simulink model "WindFarmGFMControlFast"  (R2023a)
settings: Solver=VariableStepAuto  StartTime=0.0  StopTime=Tsim  FixedStep=Ts  MaxStep=1  MinStep=Ts  RelTol=1e-3
PreLoadFcn:
  | run('WindFarmGFMControlParametersFast.m')
undefined symbols (not defined in the file): DiscIntNeverNeededParam, feeder, frt, gGFM, grid, line, loads, lvrt, mGFM, pmsm, time, Ts, windController, windTransformer, windTurbine
libraries: ee_lib x21, nesl_utility x14, eeGeneralControl x4, fl_lib x3, spsLeadLagFilterLib x2, eeTransforms x2, eePowerMeasurement x1, eeSinusoidalMeasurementV2 x1
(part 1 of 2)
settings Model: SimulationMode=accelerator  Creator=rajarshd  LastModifiedBy=rajarshd
settings SolverCC: MaxConsecutiveZCs=1  ZeroCrossAlgorithm=Adaptive  AutoInsertRateTranBlk=on  DecoupledContinuousIntegration=on
settings DataIOCC: ExternalInput=getinputstruct(op)  InitialState=getstatestruct(op)  SaveFormat=StructureWithTime  SaveOutput=off  DSMLogging=off  SignalLoggingName=logsWindGFMControl
settings OptimizationCC: ReuseModelBlockBuffer=off
settings DebuggingCC: IgnoredZcDiagnostic=none
settings ModelReferenceCC: EnableRefExpFcnMdlSchedulingChecks=on  EnableParallelModelReferenceBuilds=on  ParallelModelReferenceMATLABWorkerInit=Load Top Model
settings SimscapeCC: ExplicitSolverDiagnosticOptions=none  SimscapeLogType=all  SimscapeLogSimulationStatistics=on  SimscapeLogName=simlogWindFarmGFMControl  SimscapeOperatingPoint=op

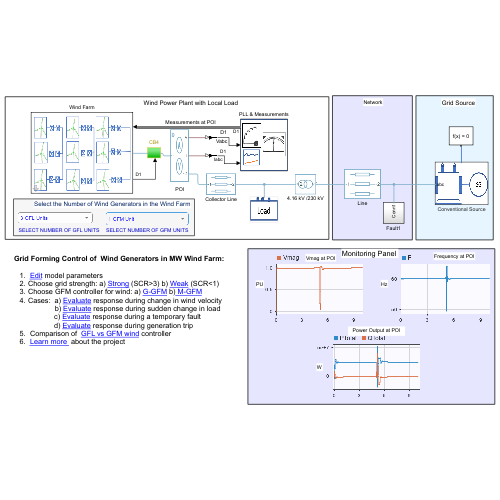
[thumbnail: Simulink's stored preview of the top-level diagram]
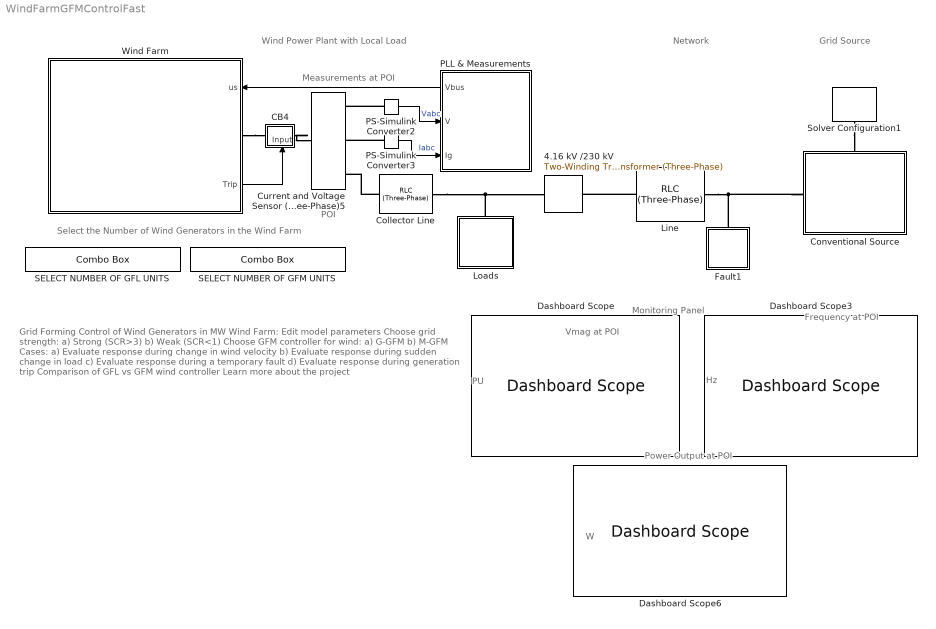
== system WindFarmGFMControlFast ==
  note: Select the Number of Wind Generators in the Wind Farm
  note: POI
  note: Measurements at POI
  note: Grid Source
  note: Wind Power Plant with Local Load
  note: Vmag at POI
  note: Frequency at POI
  note: Hz
  note: PU
  note: Grid Forming Control of Wind Generators in MW Wind Farm:
      |
      | Edit model parameters
      | Choose grid strength: a) Strong (SCR>3) b) Weak (SCR<1)
      | Choose GFM controller for wind: a) G-GFM b) M-GFM
      | Cases: a) Evaluate response during change in wind velocity
      | b) Evaluate response during sudden change in load
      | c) Evaluate response during a temporary fault
      | d) Evaluate response during generation trip
      | Comparison of GFL vs GFM wind controller
      | Learn more about the project
  note: Monitoring Panel
  note: Power Output at POI
  note: Network
  note: W
  4.16 kV /230 kV : ee_lib/Passive/Transformers/Two-Winding Transformer (Three-Phase)  SRated=windTransformer.va A*V  FRated=grid.frequency Hz  Winding1Connection=ee.enum.windingconnection.Yg  VRated1=windTransformer.hv V  Winding2Connection=ee.enum.windingconnection.Yg  VRated2=windTransformer.lv V  CoreType=ee.enum.coretype.threelimb  pu_Rw1=windTransformer.windingResistance/2  pu_Rw2=windTransformer.windingResistance/2  leakage_reactance_option=ee.enum.transformer_leakage.include  pu_Xl1=windTransformer.windingLekageReactance/2  pu_Xl2=windTransformer.windingLekageReactance/2  magnetizing_resistance_option=ee.enum.transformer_magnetizingResistance.exclude  pu_Rm=500  magnetizing_reactance_option=ee.enum.transformer_magnetizingReactance.exclude  saturation_option=ee.enum.transformer_saturation.exclude  pu_Xm=500  current_data=[0, .002, 1, 2]  magnetic_flux_data=[0, 1.2, 1.5, 1.51]  pu_X0=windTransformer.zeroSequenceReactance  i1_specify=off  i1_priority=None  i1=[0, 0, 0] A  i1_nominal_specify=off  i1_nominal_unit=A  i1_nominal_value=1  i2_specify=off  i2_priority=None  i2=[0, 0, 0] A  i2_nominal_specify=off  i2_nominal_unit=A  i2_nominal_value=1  phi_specify=off  phi_priority=None  phi=[0, 0, 0]  phi_nominal_specify=off  phi_nominal_unit=1  phi_nominal_value=1  power_dissipated_specify=off  power_dissipated_priority=None  power_dissipated=0 W  power_dissipated_nominal_specify=off  power_dissipated_nominal_unit=W  power_dissipated_nominal_value=1
      settings: InternalSimscapePortConfiguration="{\"Bottom\":[],\"Left\":[{\"id\":\"N1\",\"label\":\"~1\",\"type\":\"foundation.electrical.three_phase\"}],\"Right\":[{\"id\":\"N2\",\"label\":\"~2\",\"type\":\"foundation.electrical.three_phase\"}],\"Top\":[]}"
  CB4 : Subsystem
      settings: PortSchema="{\"entries\":[{\"content\":{\"sides\":[{\"content\":{\"connectorIds\":[\"LConn1\"]},\"type\":\"ConnectorPlacement.EquallySpacedRectSide\",\"uuid\":\"67c0f727-7c15-41c9-98df-b3c7d57498ed\"},{\"content\":{\"connectorIds\":[\"RConn1\"],\"side\":\"RIGHT\"},\"type\":\"ConnectorPlacement.EquallySpacedRectSide\",\"uuid\":\"7fc39429-ba61-416d-b42b-93e81eb2f426\"},{\"content\":{\"side\":\"TOP\"},\"type\":\"ConnectorPlacement.EquallySpacedRectSide\",\"uuid\":\"c6dd9263-b57a-4cff-a218-af99f2798f29\"},{\"content\":{\"connectorIds\":[\"In1\"],\"side\":\"BOTTOM\"},\"type\":\"ConnectorPlacement.EquallySpacedRectSide\",\"uuid\":\"e2a2ba44-d59d-4e27-adf1-3f94e828ca78\"}]},\"type\":\"ConnectorPlacement.EquallySpacedConnector\",\"uuid\":\"b349a99b-c902-4df9-9c99-34841afb28dd\"}],\"packageUris\":[\"http://schema.mathworks.com/mf0/Connector/R2020b\"],\"version\":\"1.0\"}"
  Collector Line : ee_lib/Passive/RLC Assemblies/RLC (Three-Phase)  component_structure=ee.enum.rlc.structure.SeriesRL  R=feeder.r*feeder.length Ohm  L=feeder.l*feeder.length H  C=1e-6 F  R_parasitic=0 Ohm  G_parasitic=0 1/Ohm  IL_specify=off  IL_priority=High  IL=[0, 0, 0] A  IL_nominal_specify=off  IL_nominal_unit=A  IL_nominal_value=1  VC_specify=off  VC_priority=High  VC=[0, 0, 0] V  VC_nominal_specify=off  VC_nominal_unit=V  VC_nominal_value=1
      settings: InternalSimscapePortConfiguration="{\"Bottom\":[],\"Left\":[{\"id\":\"N1\",\"label\":\"~1\",\"type\":\"foundation.electrical.three_phase\"}],\"Right\":[{\"id\":\"N2\",\"label\":\"~2\",\"type\":\"foundation.electrical.three_phase\"}],\"Top\":[]}"
  Conventional Source : Subsystem
      settings: PortSchema="{\"entries\":[{\"content\":{\"sides\":[{\"content\":{\"connectorIds\":[\"LConn1\"]},\"type\":\"ConnectorPlacement.EquallySpacedRectSide\",\"uuid\":\"88e24179-6079-4110-b6c8-07285d357c8a\"},{\"content\":{\"connectorIds\":[],\"side\":\"RIGHT\"},\"type\":\"ConnectorPlacement.EquallySpacedRectSide\",\"uuid\":\"8f4b6582-111e-4598-90a5-fa5f81c444ee\"},{\"content\":{\"connectorIds\":[\"LConn2\"],\"side\":\"TOP\"},\"type\":\"ConnectorPlacement.EquallySpacedRectSide\",\"uuid\":\"53212e71-0f3c-4549-bc92-047e88eae9b6\"},{\"content\":{\"connectorIds\":[],\"side\":\"BOTTOM\"},\"type\":\"ConnectorPlacement.EquallySpacedRectSide\",\"uuid\":\"0193069a-d0a5-4b89-8f2a-3f6fb986b7f7\"}]},\"type\":\"ConnectorPlacement.EquallySpacedConnector\",\"uuid\":\"b2543555-7807-483c-9e73-a2cd2a98a3a5\"}],\"packageUris\":[\"http://schema.mathworks.com/mf0/Connector/R2020b\"],\"version\":\"1.0\"}"
      mask Display: image('$imagefile'); % Use "Edit Image" on toolstrip to change.
  Current and Voltage Sensor (Three-Phase)5 : ee_lib/Sensors & Transducers/Current and Voltage Sensor (Three-Phase)  vMeasurementType=ee.enum.vmeasurement.lg  outputUnit=ee.enum.unit.pu  SRated=base.mVA A*V  VRated=base.kV V  I_specify=off  I_priority=None  I=[0, 0, 0] A  I_nominal_specify=off  I_nominal_unit=A  I_nominal_value=1  V_specify=off  V_priority=None  V=[0, 0, 0] V  V_nominal_specify=off  V_nominal_unit=V  V_nominal_value=1
      settings: InternalSimscapePortConfiguration="{\"Bottom\":[],\"Left\":[{\"id\":\"N1\",\"label\":\"~1\",\"type\":\"foundation.electrical.three_phase\"}],\"Right\":[{\"id\":\"V_output\",\"label\":\"V\",\"type\":\"output\"},{\"id\":\"I_output\",\"label\":\"I\",\"type\":\"output\"},{\"id\":\"N2\",\"label\":\"~2\",\"type\":\"foundation.electrical.three_phase\"}],\"Top\":[]}"
  Dashboard Scope : DashboardScope  Ymin=-0.6  Ymax=1.1
  Dashboard Scope3 : DashboardScope  Ymin=50  Ymax=80
  Dashboard Scope6 : DashboardScope
  Fault1 : Subsystem
      settings: PortSchema="{\"entries\":[{\"content\":{\"sides\":[{\"content\":{},\"type\":\"ConnectorPlacement.EquallySpacedRectSide\",\"uuid\":\"8f0a92ab-8e67-482c-af4d-aec2c4f39f54\"},{\"content\":{\"side\":\"RIGHT\"},\"type\":\"ConnectorPlacement.EquallySpacedRectSide\",\"uuid\":\"ef292762-0220-4a9e-ab1f-c2e04fa471eb\"},{\"content\":{\"connectorIds\":[\"LConn1\"],\"side\":\"TOP\"},\"type\":\"ConnectorPlacement.EquallySpacedRectSide\",\"uuid\":\"ae2b4012-1172-468f-8626-eed330b859d8\"}]},\"type\":\"ConnectorPlacement.EquallySpacedConnector\",\"uuid\":\"c563c82f-8ad7-4cb2-b357-8e612dcbe120\"}],\"packageUris\":[\"http://schema.mathworks.com/mf0/Connector/R2020b\"],\"version\":\"1.0\"}"
  Line : ee_lib/Passive/RLC Assemblies/RLC (Three-Phase)  component_structure=ee.enum.rlc.structure.SeriesRL  R=line.r*line.length1 Ohm  L=line.l*line.length1 mH  C=1e-6 F  R_parasitic=0 Ohm  G_parasitic=0 1/Ohm  IL_specify=off  IL_priority=High  IL=[0, 0, 0] A  IL_nominal_specify=off  IL_nominal_unit=A  IL_nominal_value=1  VC_specify=off  VC_priority=High  VC=[0, 0, 0] V  VC_nominal_specify=off  VC_nominal_unit=V  VC_nominal_value=1
      settings: InternalSimscapePortConfiguration="{\"Bottom\":[],\"Left\":[{\"id\":\"N1\",\"label\":\"~1\",\"type\":\"foundation.electrical.three_phase\"}],\"Right\":[{\"id\":\"N2\",\"label\":\"~2\",\"type\":\"foundation.electrical.three_phase\"}],\"Top\":[]}"
  Loads : Subsystem
      mask Display: image('$imagefile'); % Use "Edit Image" on toolstrip to change.
  PLL & Measurements : Subsystem
      settings: PortSchema="{\"entries\":[{\"content\":{\"sides\":[{\"content\":{\"connectorIds\":[\"Out1\",\"In1\",\"In2\"]},\"type\":\"ConnectorPlacement.EquallySpacedRectSide\",\"uuid\":\"76485780-20fe-4fcf-8224-69648da6ed2a\"},{\"content\":{\"side\":\"RIGHT\"},\"type\":\"ConnectorPlacement.EquallySpacedRectSide\",\"uuid\":\"f19a6390-e634-42c7-8d46-4cd80cbab182\"},{\"content\":{\"side\":\"TOP\"},\"type\":\"ConnectorPlacement.EquallySpacedRectSide\",\"uuid\":\"87682f72-1844-428e-be70-ad7ca3191ee3\"}]},\"type\":\"ConnectorPlacement.EquallySpacedConnector\",\"uuid\":\"f2136b07-48ec-402b-adb3-18c0bac2157c\"}],\"packageUris\":[\"http://schema.mathworks.com/mf0/Connector/R2020b\"],\"version\":\"1.0\"}"
      mask Display: image('measurements.png'); % Use "Edit Image" on toolstrip to change.
  PS-Simulink Converter2 : nesl_utility/PS-Simulink Converter  PhysicalDomain=network_engine_domain  SubClassName=ps_output  LeftPortType=input  RightPortType=output  PseudoPeriodic=off  Frequencies=[]  VectorFormat=inherit  Unit=inherit  AffineConversion=off
  PS-Simulink Converter3 : nesl_utility/PS-Simulink Converter  PhysicalDomain=network_engine_domain  SubClassName=ps_output  LeftPortType=input  RightPortType=output  PseudoPeriodic=off  Frequencies=[]  VectorFormat=inherit  Unit=inherit  AffineConversion=off
  SELECT NUMBER OF GFL UNITS : ComboBox  LabelPosition=Hide  SelectedLabel=3 GFL Units
      settings: Values={{'1 GFL Unit', '2 GFL Units', '3 GFL Units', '4 GFL Units', '5 GFL Units', '6 GFL Units', '7 GFL Units'}, [1 2 3 4 5 6 7]}
  SELECT NUMBER OF GFM UNITS : ComboBox  LabelPosition=Hide  SelectedLabel=1 GFM Unit  Opacity=0
      settings: Values={{'1 GFM Unit', '2 GFM Units', 'No GFM Units'}, [1 2 0]}
  Solver Configuration1 : nesl_utility/Solver Configuration  PhysicalDomain=network_engine_domain  SubClassName=solver  LeftPortType=input  RightPortType=generic  Tones=[]  Harmonics=[]  SimulateNoise=off  Profile=off  UseLocalSampling=off  EnableSwitchedLinearOptims=on  FrequencyDomain=off  UseCCode=off  RelTol=0.001  AbsTol=1e-06  MinStep=1e-09  ToWorkspace=off  RevertToSquareIcSolve=off  NumHomotopyIterations=100  PhasorMode=off  PhasorModeNumHarmonics=1  ConsistencySolver=NEWTON_FTOL  IndexReductionMethod=DerivativeReplacement  DoDC=off  ResidualTolerance=1e-3  ConsistencyTolSource=GLOBAL  ConsistencyAbsTol=0.001  ConsistencyRelTol=0.001  ConsistencyTolFactor=0.001  UseLocalSolver=on  LocalSolverChoice=NE_PARTITIONING_ADVANCER  ResolveIndetEquations=on  FunctionEvalNumThread=1  LocalSolverSampleTime=T  DoFixedCost=on  MaxNonlinIter=3  MaxModeIter=2  ComputeImpulses=off  ImpulseIterations=2  LinearAlgebra=auto  LinearAlgebraNumThread=0  EquationFormulation=NE_TIME_EF  DelaysMemoryBudget=1024  AutomaticFiltering=on  FilteringTimeConstant=0.001  PartitionStorageMethod=AS_NEEDED  PartitionMemoryBudget=1024  PartitionMethod=ROBUST
  Wind Farm : Subsystem  mask{nGFL=3, nGFM=1}
      mask prompts: nGFL "Number of GFL Wind Generators"; nGFM "Number of GFM Wind Turbines"
      settings: PortSchema="{\"entries\":[{\"content\":{\"sides\":[{\"content\":{\"connectorIds\":[\"In1\",\"LConn1\",\"Out1\"]},\"type\":\"ConnectorPlacement.EquallySpacedRectSide\",\"uuid\":\"1189e956-e6f0-4ada-905a-6b9abec668a8\"},{\"content\":{\"side\":\"RIGHT\"},\"type\":\"ConnectorPlacement.EquallySpacedRectSide\",\"uuid\":\"3ddb8f28-1c9c-423f-814f-a5e5ca919d79\"},{\"content\":{\"side\":\"TOP\"},\"type\":\"ConnectorPlacement.EquallySpacedRectSide\",\"uuid\":\"c360f229-efd7-488e-97f8-90fd9e6e05d4\"},{\"content\":{\"side\":\"BOTTOM\"},\"type\":\"ConnectorPlacement.EquallySpacedRectSide\",\"uuid\":\"99811ca4-1621-4e62-9767-ce3bd58f839c\"}]},\"type\":\"ConnectorPlacement.EquallySpacedConnector\",\"uuid\":\"16843f42-9f9b-4252-a0c2-a64badb15c83\"}],\"packageUris\":[\"http://schema.mathworks.com/mf0/Connector/R2020b\"],\"version\":\"1.0\"}"
      mask TypeOptions nGFL: 1 | 2 | 3 | 4 | 5 | 6 | 7
      mask TypeOptions nGFM: 0 | 1 | 2
      mask DialogControl Control1 Prompt: This is a Wind Farm with type-4 GFL and GFM Wind Turbine Generators
      mask Display: image('$imagefile'); % Use "Edit Image" on toolstrip to change.
  wires:
  PS-Simulink Converter2/1 -> PLL & Measurements/1(V)  "Vabc"
  PS-Simulink Converter3/1 -> PLL & Measurements/2(Ig)  "Iabc"
  PLL & Measurements/1(Vbus) -> Wind Farm/1(us)
  Wind Farm/1(Trip) -> CB4/1(Input)
  connections:
  Loads/RConn1 -- Collector Line/RConn1 -- 4.16 kV /230 kV/RConn1
  PS-Simulink Converter2/LConn1 -- Current and Voltage Sensor (Three-Phase)5/RConn1
  PS-Simulink Converter3/LConn1 -- Current and Voltage Sensor (Three-Phase)5/RConn2
  Solver Configuration1/RConn1 -- Conventional Source/LConn2
  CB4/RConn1 -- Current and Voltage Sensor (Three-Phase)5/LConn1
  Conventional Source/LConn1 -- Line/RConn1 -- Fault1/LConn1
  Line/LConn1 -- 4.16 kV /230 kV/LConn1
  Wind Farm/LConn1 -- CB4/LConn1
  Collector Line/LConn1 -- Current and Voltage Sensor (Three-Phase)5/RConn3

== system WindFarmGFMControlFast/CB4 ==
  Input : Inport
  Circuit Breaker Step off3 : ee_lib/Switches & Breakers/Circuit Breaker (Three-Phase)  R_closed=0.001 Ohm  G_open=1e-4 1/Ohm  threshold=0.5 V  breaker_behavior=ee.enum.switches.breakerBehavior.zeroCrossingEnable
      settings: InternalSimscapePortConfiguration="{\"Bottom\":[],\"Left\":[{\"id\":\"vT\",\"label\":\"vT\",\"type\":\"input\"},{\"id\":\"N1\",\"label\":\"~1\",\"type\":\"foundation.electrical.three_phase\"}],\"Right\":[{\"id\":\"N2\",\"label\":\"~2\",\"type\":\"foundation.electrical.three_phase\"}],\"Top\":[]}"
  Simulink-PS Converter3 : nesl_utility/Simulink-PS Converter  PhysicalDomain=network_engine_domain  SubClassName=ps_input  LeftPortType=input  RightPortType=output  PseudoPeriodic=off  Frequencies=[]  NoiseDistribution=none  NoiseParameters=[]  Unit=1  AffineConversion=off  FilteringAndDerivatives=zero  SimscapeFilterOrder=1  InputFilterTimeConstant=0.001  UdotUserProvided=1
  Conn2 : PMIOPort  Side=Left
  Conn1 : PMIOPort  Port=2  Side=Right
  wires:
  Input/1 -> Simulink-PS Converter3/1
  connections:
  Circuit Breaker Step off3/LConn2 -- Conn2/RConn1
  Circuit Breaker Step off3/LConn1 -- Simulink-PS Converter3/RConn1
  Circuit Breaker Step off3/RConn1 -- Conn1/RConn1

== system WindFarmGFMControlFast/Conventional Source ==
  Current and Voltage Sensor (Three-Phase)4 : ee_lib/Sensors & Transducers/Current and Voltage Sensor (Three-Phase)  vMeasurementType=ee.enum.vmeasurement.lg  outputUnit=ee.enum.unit.si  SRated=base.mVA A*V  VRated=base.kV V  I_specify=off  I_priority=None  I=[0, 0, 0] A  I_nominal_specify=off  I_nominal_unit=A  I_nominal_value=1  V_specify=off  V_priority=None  V=[0, 0, 0] V  V_nominal_specify=off  V_nominal_unit=V  V_nominal_value=1
      settings: InternalSimscapePortConfiguration="{\"Bottom\":[],\"Left\":[{\"id\":\"N1\",\"label\":\"~1\",\"type\":\"foundation.electrical.three_phase\"}],\"Right\":[{\"id\":\"V_output\",\"label\":\"V\",\"type\":\"output\"},{\"id\":\"I_output\",\"label\":\"I\",\"type\":\"output\"},{\"id\":\"N2\",\"label\":\"~2\",\"type\":\"foundation.electrical.three_phase\"}],\"Top\":[]}"
  Frequency Controlled Source : Subsystem  VariantControl=VSMFrequencyControlledSource
  Measurements : Subsystem
  PS-Simulink Converter2 : nesl_utility/PS-Simulink Converter  PhysicalDomain=network_engine_domain  SubClassName=ps_output  LeftPortType=input  RightPortType=output  PseudoPeriodic=off  Frequencies=[]  VectorFormat=inherit  Unit=inherit  AffineConversion=off
  PS-Simulink Converter3 : nesl_utility/PS-Simulink Converter  PhysicalDomain=network_engine_domain  SubClassName=ps_output  LeftPortType=input  RightPortType=output  PseudoPeriodic=off  Frequencies=[]  VectorFormat=inherit  Unit=inherit  AffineConversion=off
  abc : PMIOPort  Side=Left
  Connection Port : PMIOPort  Port=2  Side=Left
  wires:
  PS-Simulink Converter3/1 -> Measurements/2(I)
  Measurements/1(Grid) -> Frequency Controlled Source/1(Grid)
  PS-Simulink Converter2/1 -> Measurements/1(V)
  connections:
  Current and Voltage Sensor (Three-Phase)4/RConn3 -- abc/RConn1
  PS-Simulink Converter2/LConn1 -- Current and Voltage Sensor (Three-Phase)4/RConn1
  PS-Simulink Converter3/LConn1 -- Current and Voltage Sensor (Three-Phase)4/RConn2
  Frequency Controlled Source/RConn1 -- Current and Voltage Sensor (Three-Phase)4/LConn1
  Frequency Controlled Source/LConn1 -- Connection Port/RConn1

== system WindFarmGFMControlFast/Fault1 ==
  CB1 : Subsystem
      settings: PortSchema="{\"entries\":[{\"content\":{\"sides\":[{\"content\":{\"connectorIds\":[\"LConn1\"]},\"type\":\"ConnectorPlacement.EquallySpacedRectSide\",\"uuid\":\"67c0f727-7c15-41c9-98df-b3c7d57498ed\"},{\"content\":{\"connectorIds\":[\"RConn1\"],\"side\":\"RIGHT\"},\"type\":\"ConnectorPlacement.EquallySpacedRectSide\",\"uuid\":\"7fc39429-ba61-416d-b42b-93e81eb2f426\"},{\"content\":{\"connectorIds\":[],\"side\":\"TOP\"},\"type\":\"ConnectorPlacement.EquallySpacedRectSide\",\"uuid\":\"c6dd9263-b57a-4cff-a218-af99f2798f29\"},{\"content\":{\"connectorIds\":[\"In1\"],\"side\":\"BOTTOM\"},\"type\":\"ConnectorPlacement.EquallySpacedRectSide\",\"uuid\":\"e2a2ba44-d59d-4e27-adf1-3f94e828ca78\"}]},\"type\":\"ConnectorPlacement.EquallySpacedConnector\",\"uuid\":\"b349a99b-c902-4df9-9c99-34841afb28dd\"}],\"packageUris\":[\"http://schema.mathworks.com/mf0/Connector/R2020b\"],\"version\":\"1.0\"}"
  Fault : ee_lib/Passive/RLC Assemblies/RLC (Three-Phase)  component_structure=ee.enum.rlc.structure.SeriesRL  R=1e-4 Ohm  L=1e-4 mH  C=1e-6 F  R_parasitic=0 Ohm  G_parasitic=1e-4 1/Ohm  IL_specify=off  IL_priority=High  IL=[0, 0, 0] A  IL_nominal_specify=off  IL_nominal_unit=A  IL_nominal_value=1  VC_specify=off  VC_priority=High  VC=[0, 0, 0] V  VC_nominal_specify=off  VC_nominal_unit=V  VC_nominal_value=1
      settings: InternalSimscapePortConfiguration="{\"Bottom\":[],\"Left\":[{\"id\":\"N1\",\"label\":\"~1\",\"type\":\"foundation.electrical.three_phase\"}],\"Right\":[{\"id\":\"N2\",\"label\":\"~2\",\"type\":\"foundation.electrical.three_phase\"}],\"Top\":[]}"
  Grounded Neutral (Three-Phase) : ee_lib/Connectors & References/Grounded Neutral (Three-Phase)
  Step1 : Step  Time=time.fault+0.140  SampleTime=Ts
  Step2 : Step  Time=time.fault  Before=1  After=0  SampleTime=Ts
  Sum : Sum  Inputs=|++
  Conn1 : PMIOPort  Side=Left
  wires:
  Step1/1 -> Sum/2
  Sum/1 -> CB1/1(Input)
  Step2/1 -> Sum/1
  connections:
  CB1/RConn1 -- Fault/LConn1
  CB1/LConn1 -- Conn1/RConn1
  Grounded Neutral (Three-Phase)/LConn1 -- Fault/RConn1

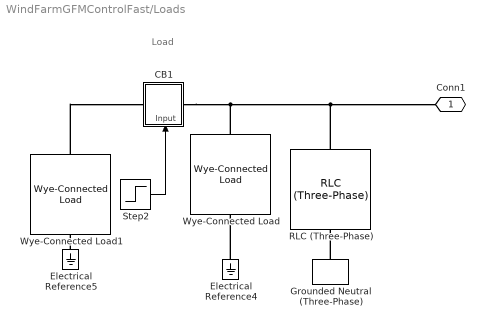
== system WindFarmGFMControlFast/Loads ==
  note: Load
  CB1 : Subsystem
      settings: PortSchema="{\"entries\":[{\"content\":{\"sides\":[{\"content\":{\"connectorIds\":[\"LConn1\"]},\"type\":\"ConnectorPlacement.EquallySpacedRectSide\",\"uuid\":\"67c0f727-7c15-41c9-98df-b3c7d57498ed\"},{\"content\":{\"connectorIds\":[\"RConn1\"],\"side\":\"RIGHT\"},\"type\":\"ConnectorPlacement.EquallySpacedRectSide\",\"uuid\":\"7fc39429-ba61-416d-b42b-93e81eb2f426\"},{\"content\":{\"connectorIds\":[],\"side\":\"TOP\"},\"type\":\"ConnectorPlacement.EquallySpacedRectSide\",\"uuid\":\"c6dd9263-b57a-4cff-a218-af99f2798f29\"},{\"content\":{\"connectorIds\":[\"In1\"],\"side\":\"BOTTOM\"},\"type\":\"ConnectorPlacement.EquallySpacedRectSide\",\"uuid\":\"e2a2ba44-d59d-4e27-adf1-3f94e828ca78\"}]},\"type\":\"ConnectorPlacement.EquallySpacedConnector\",\"uuid\":\"b349a99b-c902-4df9-9c99-34841afb28dd\"}],\"packageUris\":[\"http://schema.mathworks.com/mf0/Connector/R2020b\"],\"version\":\"1.0\"}"
  Electrical Reference4 : fl_lib/Electrical/Electrical Elements/Electrical Reference
  Electrical Reference5 : fl_lib/Electrical/Electrical Elements/Electrical Reference
  Grounded Neutral (Three-Phase) : ee_lib/Connectors & References/Grounded Neutral (Three-Phase)
  RLC (Three-Phase) : ee_lib/Passive/RLC Assemblies/RLC (Three-Phase)  component_structure=ee.enum.rlc.structure.C  R=feeder.r*0.01 Ohm  L=feeder.l*0.01 H  C=1e-6 F  R_parasitic=0 Ohm  G_parasitic=0 1/Ohm  IL_specify=off  IL_priority=High  IL=[0, 0, 0] A  IL_nominal_specify=off  IL_nominal_unit=A  IL_nominal_value=1  VC_specify=off  VC_priority=High  VC=[0, 0, 0] V  VC_nominal_specify=off  VC_nominal_unit=V  VC_nominal_value=1
      settings: InternalSimscapePortConfiguration="{\"Bottom\":[],\"Left\":[{\"id\":\"N1\",\"label\":\"~1\",\"type\":\"foundation.electrical.three_phase\"}],\"Right\":[{\"id\":\"N2\",\"label\":\"~2\",\"type\":\"foundation.electrical.three_phase\"}],\"Top\":[]}"
  Step2 : Step  Time=time.load  Before=1  After=0  SampleTime=Ts
  Wye-Connected Load : ee_lib/Passive/RLC Assemblies/Wye-Connected Load  parameterization=ee.enum.rlc.parameterization.ratedpower  component_structure=ee.enum.rlc.structure.R  component_structure_PQ=ee.enum.rlc.structure.R  R=1 Ohm  L=1e-3 H  C=1e-6 F  VRated=windTransformer.lv V  FRated=60 Hz  P=loads.P2 W  Qpos=1e2 A*V  Qneg=-1e2 A*V  R_parasitic=0 Ohm  G_parasitic=0 1/Ohm  R_parasitic_PQ=0 Ohm  G_parasitic_PQ=0 1/Ohm  Vmag0=24e3 V  Vang0=0 deg  Freq0=60 Hz  IL_specify=off  IL_priority=High  IL=[0, 0, 0] A  IL_nominal_specify=off  IL_nominal_unit=A  IL_nominal_value=1  VC_specify=off  VC_priority=High  VC=[0, 0, 0] V  VC_nominal_specify=off  VC_nominal_unit=V  VC_nominal_value=1
  Wye-Connected Load1 : ee_lib/Passive/RLC Assemblies/Wye-Connected Load  parameterization=ee.enum.rlc.parameterization.ratedpower  component_structure=ee.enum.rlc.structure.R  component_structure_PQ=ee.enum.rlc.structure.R  R=1 Ohm  L=1e-3 H  C=1e-6 F  VRated=windTransformer.lv V  FRated=60 Hz  P=loads.P1 W  Qpos=loads.Q1 A*V  Qneg=-1e2 A*V  R_parasitic=0 Ohm  G_parasitic=0 1/Ohm  R_parasitic_PQ=0 Ohm  G_parasitic_PQ=0 1/Ohm  Vmag0=24e3 V  Vang0=0 deg  Freq0=60 Hz  IL_specify=off  IL_priority=High  IL=[0, 0, 0] A  IL_nominal_specify=off  IL_nominal_unit=A  IL_nominal_value=1  VC_specify=off  VC_priority=High  VC=[0, 0, 0] V  VC_nominal_specify=off  VC_nominal_unit=V  VC_nominal_value=1
  Conn1 : PMIOPort  Side=Right
  wires:
  Step2/1 -> CB1/1(Input)
  connections:
  Electrical Reference4/LConn1 -- Wye-Connected Load/RConn1
  Wye-Connected Load1/LConn1 -- CB1/LConn1
  CB1/RConn1 -- Wye-Connected Load/LConn1 -- RLC (Three-Phase)/LConn1 -- Conn1/RConn1
  Electrical Reference5/LConn1 -- Wye-Connected Load1/RConn1
  Grounded Neutral (Three-Phase)/LConn1 -- RLC (Three-Phase)/RConn1

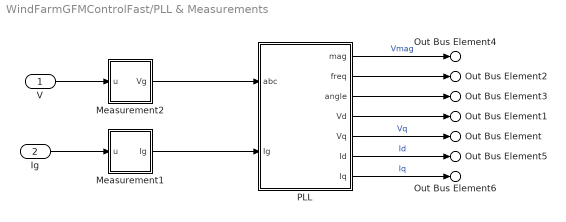
== system WindFarmGFMControlFast/PLL & Measurements ==
  V : Inport
  Ig : Inport  Port=2
  Measurement1 : Subsystem
  Measurement2 : Subsystem
  PLL : Subsystem
  Out Bus Element : Outport  PortName=Vbus  Element=Vq
  Out Bus Element1 : Outport  PortName=Vbus  Element=Vd
  Out Bus Element2 : Outport  PortName=Vbus  Element=w
  Out Bus Element3 : Outport  PortName=Vbus  Element=Theta
  Out Bus Element4 : Outport  PortName=Vbus  Element=Vmag
  Out Bus Element5 : Outport  PortName=Vbus  Element=Id
  Out Bus Element6 : Outport  PortName=Vbus  Element=Iq
  wires:
  V/1 -> Measurement2/1(u)
  PLL/2(freq) -> Out Bus Element2/1
  PLL/5(Vq) -> Out Bus Element/1  "Vq"
  PLL/3(angle) -> Out Bus Element3/1
  PLL/4(Vd) -> Out Bus Element1/1
  Measurement2/1(Vg) -> PLL/1(abc)
  PLL/1(mag) -> Out Bus Element4/1  "Vmag"
  Measurement1/1(Ig) -> PLL/2(Ig)
  Ig/1 -> Measurement1/1(u)
  PLL/7(Iq) -> Out Bus Element6/1  "Iq"
  PLL/6(Id) -> Out Bus Element5/1  "Id"

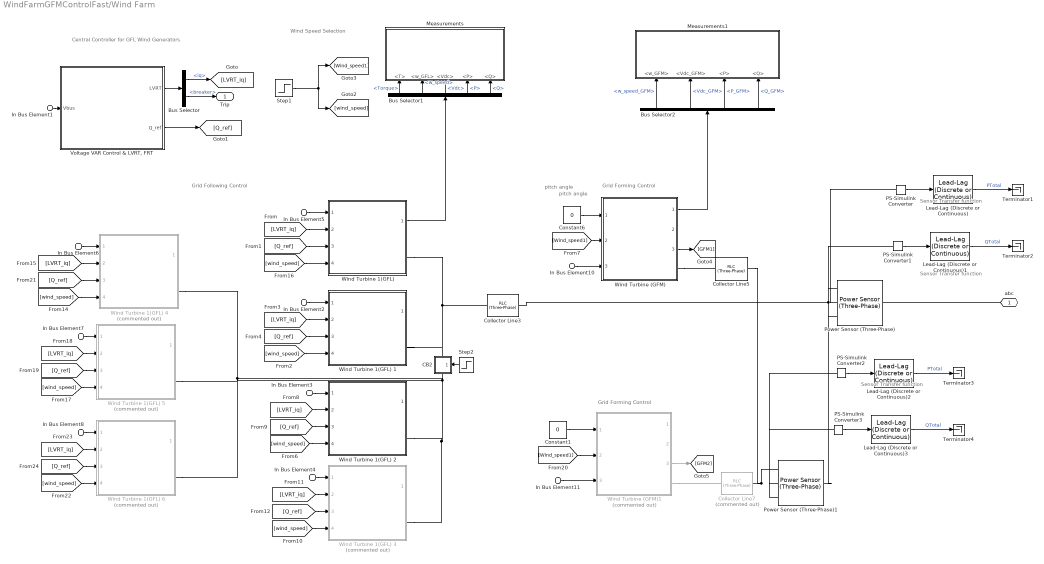
== system WindFarmGFMControlFast/Wind Farm ==
  note: Sensor Transfer function
  note: Central Controller for GFL Wind Generators
  note: Wind Speed Selection
  note: Sensor Transfer function
  note: pitch angle
  note: Grid Following Control
  note: Grid Forming Control
  note: Grid Forming Control
  note: pitch angle
  note: Sensor Transfer function
  In Bus Element{1..8,10..11} (10 alike) : Inport  PortName=us
  Bus Selector : BusSelector  OutputSignals=iq,breaker
  Bus Selector1 : BusSelector  OutputSignals=Torque,w_speed,Vdc,P,Q
  Bus Selector2 : BusSelector  OutputSignals=w_speed_GFM,Vdc_GFM,P_GFM,Q_GFM
  CB2 : Subsystem
      settings: PortSchema="{\"entries\":[{\"content\":{\"sides\":[{\"content\":{\"connectorIds\":[\"LConn1\"]},\"type\":\"ConnectorPlacement.EquallySpacedRectSide\",\"uuid\":\"67c0f727-7c15-41c9-98df-b3c7d57498ed\"},{\"content\":{\"connectorIds\":[\"RConn1\"],\"side\":\"RIGHT\"},\"type\":\"ConnectorPlacement.EquallySpacedRectSide\",\"uuid\":\"7fc39429-ba61-416d-b42b-93e81eb2f426\"},{\"content\":{\"side\":\"TOP\"},\"type\":\"ConnectorPlacement.EquallySpacedRectSide\",\"uuid\":\"c6dd9263-b57a-4cff-a218-af99f2798f29\"},{\"content\":{\"connectorIds\":[\"In1\"],\"side\":\"BOTTOM\"},\"type\":\"ConnectorPlacement.EquallySpacedRectSide\",\"uuid\":\"e2a2ba44-d59d-4e27-adf1-3f94e828ca78\"}]},\"type\":\"ConnectorPlacement.EquallySpacedConnector\",\"uuid\":\"b349a99b-c902-4df9-9c99-34841afb28dd\"}],\"packageUris\":[\"http://schema.mathworks.com/mf0/Connector/R2020b\"],\"version\":\"1.0\"}"
  Collector Line3 : ee_lib/Passive/RLC Assemblies/RLC (Three-Phase)  component_structure=ee.enum.rlc.structure.SeriesRL  R=feeder.r*0.5 Ohm  L=feeder.l*0.5 H  C=1e-6 F  R_parasitic=0 Ohm  G_parasitic=0 1/Ohm  IL_specify=off  IL_priority=High  IL=[0, 0, 0] A  IL_nominal_specify=off  IL_nominal_unit=A  IL_nominal_value=1  VC_specify=off  VC_priority=High  VC=[0, 0, 0] V  VC_nominal_specify=off  VC_nominal_unit=V  VC_nominal_value=1
      settings: InternalSimscapePortConfiguration="{\"Bottom\":[],\"Left\":[{\"id\":\"N1\",\"label\":\"~1\",\"type\":\"foundation.electrical.three_phase\"}],\"Right\":[{\"id\":\"N2\",\"label\":\"~2\",\"type\":\"foundation.electrical.three_phase\"}],\"Top\":[]}"
  Collector Line5 : ee_lib/Passive/RLC Assemblies/RLC (Three-Phase)  component_structure=ee.enum.rlc.structure.SeriesRL  R=feeder.r*0.01 Ohm  L=feeder.l*0.01 H  C=1e-6 F  R_parasitic=0 Ohm  G_parasitic=0 1/Ohm  IL_specify=off  IL_priority=High  IL=[0, 0, 0] A  IL_nominal_specify=off  IL_nominal_unit=A  IL_nominal_value=1  VC_specify=off  VC_priority=High  VC=[0, 0, 0] V  VC_nominal_specify=off  VC_nominal_unit=V  VC_nominal_value=1
      settings: InternalSimscapePortConfiguration="{\"Bottom\":[],\"Left\":[{\"id\":\"N1\",\"label\":\"~1\",\"type\":\"foundation.electrical.three_phase\"}],\"Right\":[{\"id\":\"N2\",\"label\":\"~2\",\"type\":\"foundation.electrical.three_phase\"}],\"Top\":[]}"
  Collector Line7 : ee_lib/Passive/RLC Assemblies/RLC (Three-Phase)  Commented=on  component_structure=ee.enum.rlc.structure.SeriesRL  R=feeder.r*0.01 Ohm  L=feeder.l*0.01 H  C=1e-6 F  R_parasitic=0 Ohm  G_parasitic=0 1/Ohm  IL_specify=off  IL_priority=High  IL=[0, 0, 0] A  IL_nominal_specify=off  IL_nominal_unit=A  IL_nominal_value=1  VC_specify=off  VC_priority=High  VC=[0, 0, 0] V  VC_nominal_specify=off  VC_nominal_unit=V  VC_nominal_value=1
      settings: InternalSimscapePortConfiguration="{\"Bottom\":[],\"Left\":[{\"id\":\"N1\",\"label\":\"~1\",\"type\":\"foundation.electrical.three_phase\"}],\"Right\":[{\"id\":\"N2\",\"label\":\"~2\",\"type\":\"foundation.electrical.three_phase\"}],\"Top\":[]}"
  Constant1 : Constant  Value=0
  Constant6 : Constant  Value=0
  Lead-Lag (Discrete or Continuous){,1..3} (4 alike) : eeGeneralControl/Lead-Lag (Discrete or Continuous)  T1=0  T2=windController.tSensor  B=inf  A=-inf  init_option=Inherited from block input  x0=0  Ts=Ts
      settings: LibrarySourceBlock=|
      | ee_sl_lib/General Control/Lead-Lag
      | (Discrete or Continuous)
  Measurements : Subsystem
  Measurements1 : Subsystem
  PS-Simulink Converter{,1..3} (4 alike) : nesl_utility/PS-Simulink Converter  PhysicalDomain=network_engine_domain  SubClassName=ps_output  LeftPortType=input  RightPortType=output  PseudoPeriodic=off  Frequencies=[]  VectorFormat=inherit  Unit=inherit  AffineConversion=off
  Power Sensor (Three-Phase) : ee_lib/Sensors & Transducers/Power Sensor (Three-Phase)  load_type=ee.enum.passive.type_balanced.balanced  f0=60 Hz  config=ee.enum.with_neutral.no  rho=1
      settings: InternalSimscapePortConfiguration="{\"Bottom\":[],\"Left\":[{\"id\":\"N1\",\"label\":\"~1\",\"type\":\"foundation.electrical.three_phase\"}],\"Right\":[{\"id\":\"N2\",\"label\":\"~2\",\"type\":\"foundation.electrical.three_phase\"}],\"Top\":[{\"id\":\"Pm\",\"label\":\"P\",\"type\":\"output\"},{\"id\":\"Qm\",\"label\":\"Q\",\"type\":\"output\"}]}"
  Power Sensor (Three-Phase)1 : ee_lib/Sensors & Transducers/Power Sensor (Three-Phase)  load_type=ee.enum.passive.type_balanced.balanced  f0=60 Hz  config=ee.enum.with_neutral.no  rho=1
      settings: InternalSimscapePortConfiguration="{\"Bottom\":[],\"Left\":[{\"id\":\"N1\",\"label\":\"~1\",\"type\":\"foundation.electrical.three_phase\"}],\"Right\":[{\"id\":\"N2\",\"label\":\"~2\",\"type\":\"foundation.electrical.three_phase\"}],\"Top\":[{\"id\":\"Pm\",\"label\":\"P\",\"type\":\"output\"},{\"id\":\"Qm\",\"label\":\"Q\",\"type\":\"output\"}]}"
  Step1 : Step  Time=time.wind  Before=12  After=8  SampleTime=5e-5  ZeroCross=off
  Step2 : Step  Time=time.lineTrip  SampleTime=Ts
  Terminator{1..4} (4 alike) : Terminator
  "Voltage VAR Control & LVRT, FRT" : Subsystem
      mask Display: image('$imagefile'); % Use "Edit Image" on toolstrip to change.
  Wind Turbine (GFM) : Subsystem  ReferencedSubsystem=gfmWind  Control=VSM Using DC Link Voltage  V_ref=gGFM.vref  Q_ref=gGFM.qref  Kq=gGFM.kq  Kt=gGFM.kt  KqI=mGFM.kq  Kp=mGFM.kp  Kd=gGFM.kd  Kj=gGFM.kj  H=mGFM.h  D=mGFM.d  Vd_ref=mGFM.Vd  frequency1=gGFM.fref  frequency=mGFM.fref  x_vir=mGFM.x_vir  x_vir1=gGFM.r_vir  r_vir1=gGFM.x_vir  Imax1=gGFM.Imax  Imax=mGFM.Imax  r_vir=mGFM.r_vir  Kpq_mpp=pmsm.lq*pmsm.alpha  Kpd_mpp=pmsm.ld*pmsm.alpha  Kiq_mpp=pmsm.rs*pmsm.alpha  Kid_mpp=pmsm.rs*pmsm.alpha  Kpq=pmsm.lq*pmsm.alpha  Kpd=pmsm.ld*pmsm.alpha  Kiq=pmsm.rs*pmsm.alpha  Kid=pmsm.rs*pmsm.alpha  Kp_dc_sm=mGFM.kpdc  Ki_dc_sm=mGFM.kidc  wt1=0.01  rt1=0.01  pitch1=windTurbine.pitch  cp1=windTurbine.cp  airDensity1=windTurbine.airDensity  TSR1=windTurbine.TSR  Radius1=windTurbine.turbineRadius  wt=0.01  rt=0.01  pitch=windTurbine.pitch  cp=windTurbine.cp  airDensity=windTurbine.airDensity  Radius=windTurbine.turbineRadius  TSR=windTurbine.TSR  Inertia1=windTurbine.inertia  Inertia=windTurbine.inertia  psim1=pmsm.psim  p1=pmsm.p  Rs1=pmsm.rs  Lq1=pmsm.lq  Ld1=pmsm.ld  Ld=pmsm.ld  Lq=pmsm.lq  Rs=pmsm.rs  p=pmsm.p  psim=pmsm.psim
  Wind Turbine (GFM)1 : Subsystem  Commented=on  ReferencedSubsystem=gfmWind  Control=VSM Using DC Link Voltage  V_ref=gGFM.vref  Q_ref=gGFM.qref  Kq=gGFM.kq  Kt=gGFM.kt  KqI=mGFM.kq  Kp=mGFM.kp  Kd=gGFM.kd  Kj=gGFM.kj  H=mGFM.h  D=mGFM.d  Vd_ref=mGFM.Vd  frequency1=gGFM.fref  frequency=mGFM.fref  x_vir=mGFM.x_vir  x_vir1=gGFM.r_vir  r_vir1=gGFM.x_vir  Imax1=gGFM.Imax  Imax=mGFM.Imax  r_vir=mGFM.r_vir  Kpq_mpp=pmsm.lq*pmsm.alpha  Kpd_mpp=pmsm.ld*pmsm.alpha  Kiq_mpp=pmsm.rs*pmsm.alpha  Kid_mpp=pmsm.rs*pmsm.alpha  Kpq=pmsm.lq*pmsm.alpha  Kpd=pmsm.ld*pmsm.alpha  Kiq=pmsm.rs*pmsm.alpha  Kid=pmsm.rs*pmsm.alpha  Kp_dc_sm=mGFM.kpdc  Ki_dc_sm=mGFM.kidc  wt1=0.01  rt1=0.01  pitch1=windTurbine.pitch  cp1=windTurbine.cp  airDensity1=windTurbine.airDensity  TSR1=windTurbine.TSR  Radius1=windTurbine.turbineRadius  wt=0.01  rt=0.01  pitch=windTurbine.pitch  cp=windTurbine.cp  airDensity=windTurbine.airDensity  Radius=windTurbine.turbineRadius  TSR=windTurbine.TSR  Inertia1=windTurbine.inertia  Inertia=windTurbine.inertia  psim1=pmsm.psim  p1=pmsm.p  Rs1=pmsm.rs  Lq1=pmsm.lq  Ld1=pmsm.ld  Ld=pmsm.ld  Lq=pmsm.lq  Rs=pmsm.rs  p=pmsm.p  psim=pmsm.psim
  Wind Turbine 1(GFL) : Subsystem  ReferencedSubsystem=WindGFLMpp23a  p=pmsm.p  psim=pmsm.psim  Rs=pmsm.rs  Ld=pmsm.ld  Lq=pmsm.lq  Kdip_sm=pmsm.ld*pmsm.alpha  Kdii_sm=pmsm.rs*pmsm.alpha  Kqip_sm=pmsm.lq*pmsm.alpha  Kqii_sm=pmsm.rs*pmsm.alpha  airDensity=windTurbine.airDensity  turbineRadius=windTurbine.turbineRadius  pitch=windTurbine.pitch  TSR=windTurbine.TSR  cp=windTurbine.cp  wt=0.01  rt=0.01  Inertia=windTurbine.inertia  Kp_dc=windController.kpv  Ki_dc=windController.kiv  Kdpi_g=windController.kpic  Kdii_g=windController.kiic  Kqpi_g=windController.kpic  Kqii_g=windController.kiic
  Wind Turbine 1(GFL) 1 : Subsystem  ReferencedSubsystem=WindGFLMpp23a  p=pmsm.p  psim=pmsm.psim  Rs=pmsm.rs  Ld=pmsm.ld  Lq=pmsm.lq  Kdip_sm=pmsm.ld*pmsm.alpha  Kdii_sm=pmsm.rs*pmsm.alpha  Kqip_sm=pmsm.lq*pmsm.alpha  Kqii_sm=pmsm.rs*pmsm.alpha  airDensity=windTurbine.airDensity  turbineRadius=windTurbine.turbineRadius  pitch=windTurbine.pitch  TSR=windTurbine.TSR  cp=windTurbine.cp  wt=0.01  rt=0.01  Inertia=windTurbine.inertia  Kp_dc=windController.kpv  Ki_dc=windController.kiv  Kdpi_g=windController.kpic  Kdii_g=windController.kiic  Kqpi_g=windController.kpic  Kqii_g=windController.kiic
  Wind Turbine 1(GFL) 2 : Subsystem  ReferencedSubsystem=WindGFLMpp23a  p=pmsm.p  psim=pmsm.psim  Rs=pmsm.rs  Ld=pmsm.ld  Lq=pmsm.lq  Kdip_sm=pmsm.ld*pmsm.alpha  Kdii_sm=pmsm.rs*pmsm.alpha  Kqip_sm=pmsm.lq*pmsm.alpha  Kqii_sm=pmsm.rs*pmsm.alpha  airDensity=windTurbine.airDensity  turbineRadius=windTurbine.turbineRadius  pitch=windTurbine.pitch  TSR=windTurbine.TSR  cp=windTurbine.cp  wt=0.01  rt=0.01  Inertia=windTurbine.inertia  Kp_dc=windController.kpv  Ki_dc=windController.kiv  Kdpi_g=windController.kpic  Kdii_g=windController.kiic  Kqpi_g=windController.kpic  Kqii_g=windController.kiic
  Wind Turbine 1(GFL) {3..6} (4 alike) : Subsystem  Commented=on  ReferencedSubsystem=WindGFLMpp23a  p=pmsm.p  psim=pmsm.psim  Rs=pmsm.rs  Ld=pmsm.ld  Lq=pmsm.lq  Kdip_sm=pmsm.ld*pmsm.alpha  Kdii_sm=pmsm.rs*pmsm.alpha  Kqip_sm=pmsm.lq*pmsm.alpha  Kqii_sm=pmsm.rs*pmsm.alpha  airDensity=windTurbine.airDensity  turbineRadius=windTurbine.turbineRadius  pitch=windTurbine.pitch  TSR=windTurbine.TSR  cp=windTurbine.cp  wt=0.01  rt=0.01  Inertia=windTurbine.inertia  Kp_dc=windController.kpv  Ki_dc=windController.kiv  Kdpi_g=windController.kpic  Kdii_g=windController.kiic  Kqpi_g=windController.kpic  Kqii_g=windController.kiic
  abc : PMIOPort  Side=Left
  Trip : Outport
  wires:
  "Voltage VAR Control & LVRT, FRT"/1(LVRT) -> Bus Selector/1
  In Bus Element1/1 -> "Voltage VAR Control & LVRT, FRT"/1(Vbus)
  Bus Selector/2 -> Trip/1  "<breaker>"
  Bus Selector1/4 -> Measurements/4(<P>)  "<P>"
  Bus Selector1/5 -> Measurements/5(<Q>)  "<Q>"
  Bus Selector1/1 -> Measurements/1(<T>)  "<Torque>"
  Bus Selector1/3 -> Measurements/3(<Vdc>)  "<Vdc>"
  Bus Selector1/2 -> Measurements/2(<w_GFL>)  "<w_speed>"
  "Voltage VAR Control & LVRT, FRT"/2(Q_ref) -> [Q_ref]
  Bus Selector/1 -> [LVRT_iq]  "<iq>"
  PS-Simulink Converter1/1 -> Lead-Lag (Discrete or Continuous)1/1
  Lead-Lag (Discrete or Continuous)/1 -> Terminator1/1  "PTotal"
  PS-Simulink Converter/1 -> Lead-Lag (Discrete or Continuous)/1
  Lead-Lag (Discrete or Continuous)1/1 -> Terminator2/1  "QTotal"
  Wind Turbine 1(GFL)/1 -> Bus Selector1/1
  Wind Turbine (GFM)/3 -> [GFM1]
  Bus Selector2/4 -> Measurements1/4(<Q>)  "<Q_GFM>"
  Bus Selector2/3 -> Measurements1/3(<P>)  "<P_GFM>"
  Bus Selector2/1 -> Measurements1/1(<w_GFM>)  "<w_speed_GFM>"
  Bus Selector2/2 -> Measurements1/2(<Vdc_GFM>)  "<Vdc_GFM>"
  Wind Turbine (GFM)/1 -> Bus Selector2/1
  Step1/1 -> [Wind_speed1], [wind_speed]
  Step2/1 -> CB2/1(Input)
  In Bus Element6/1 -> Wind Turbine 1(GFL) 4/1
  [LVRT_iq] -> Wind Turbine 1(GFL) 4/2
  [Q_ref] -> Wind Turbine 1(GFL) 4/3
  [wind_speed] -> Wind Turbine 1(GFL) 4/4
  In Bus Element7/1 -> Wind Turbine 1(GFL) 5/1
  [LVRT_iq] -> Wind Turbine 1(GFL) 5/2
  [Q_ref] -> Wind Turbine 1(GFL) 5/3
  [wind_speed] -> Wind Turbine 1(GFL) 5/4
  In Bus Element8/1 -> Wind Turbine 1(GFL) 6/1
  [LVRT_iq] -> Wind Turbine 1(GFL) 6/2
  [Q_ref] -> Wind Turbine 1(GFL) 6/3
  [wind_speed] -> Wind Turbine 1(GFL) 6/4
  [LVRT_iq] -> Wind Turbine 1(GFL)/2
  In Bus Element5/1 -> Wind Turbine 1(GFL)/1
  [Q_ref] -> Wind Turbine 1(GFL)/3
  [wind_speed] -> Wind Turbine 1(GFL)/4
  In Bus Element2/1 -> Wind Turbine 1(GFL) 1/1
  [LVRT_iq] -> Wind Turbine 1(GFL) 1/2
  [Q_ref] -> Wind Turbine 1(GFL) 1/3
  [wind_speed] -> Wind Turbine 1(GFL) 1/4
  In Bus Element3/1 -> Wind Turbine 1(GFL) 2/1
  [LVRT_iq] -> Wind Turbine 1(GFL) 2/2
  [Q_ref] -> Wind Turbine 1(GFL) 2/3
  [wind_speed] -> Wind Turbine 1(GFL) 2/4
  In Bus Element4/1 -> Wind Turbine 1(GFL) 3/1
  [LVRT_iq] -> Wind Turbine 1(GFL) 3/2
  [Q_ref] -> Wind Turbine 1(GFL) 3/3
  [wind_speed] -> Wind Turbine 1(GFL) 3/4
  Constant6/1 -> Wind Turbine (GFM)/1
  [Wind_speed1] -> Wind Turbine (GFM)/2
  In Bus Element10/1 -> Wind Turbine (GFM)/3
  Constant1/1 -> Wind Turbine (GFM)1/1
  [Wind_speed1] -> Wind Turbine (GFM)1/2
  In Bus Element11/1 -> Wind Turbine (GFM)1/3
  Wind Turbine (GFM)1/3 -> [GFM2]
  PS-Simulink Converter3/1 -> Lead-Lag (Discrete or Continuous)3/1
  Lead-Lag (Discrete or Continuous)3/1 -> Terminator4/1  "QTotal"
  PS-Simulink Converter2/1 -> Lead-Lag (Discrete or Continuous)2/1
  Lead-Lag (Discrete or Continuous)2/1 -> Terminator3/1  "PTotal"
  connections:
  abc/RConn1 -- Power Sensor (Three-Phase)/RConn1
  PS-Simulink Converter/LConn1 -- Power Sensor (Three-Phase)/LConn2
  Power Sensor (Three-Phase)/LConn3 -- PS-Simulink Converter1/LConn1
  Collector Line3/RConn1 -- Power Sensor (Three-Phase)1/RConn1 -- Power Sensor (Three-Phase)/LConn1
  Wind Turbine (GFM)/RConn1 -- Collector Line5/LConn1
  Wind Turbine (GFM)1/RConn1 -- Collector Line7/LConn1
  CB2/RConn1 -- Wind Turbine 1(GFL) 1/RConn1 -- Wind Turbine 1(GFL)/RConn1 -- Collector Line3/LConn1
  Wind Turbine 1(GFL) 4/RConn1 -- Wind Turbine 1(GFL) 6/RConn1 -- Wind Turbine 1(GFL) 5/RConn1 -- Wind Turbine 1(GFL) 3/RConn1 -- Wind Turbine 1(GFL) 2/RConn1 -- CB2/LConn1
  Collector Line5/RConn1 -- Power Sensor (Three-Phase)1/LConn1 -- Collector Line7/RConn1
  Power Sensor (Three-Phase)1/LConn3 -- PS-Simulink Converter3/LConn1
  Power Sensor (Three-Phase)1/LConn2 -- PS-Simulink Converter2/LConn1

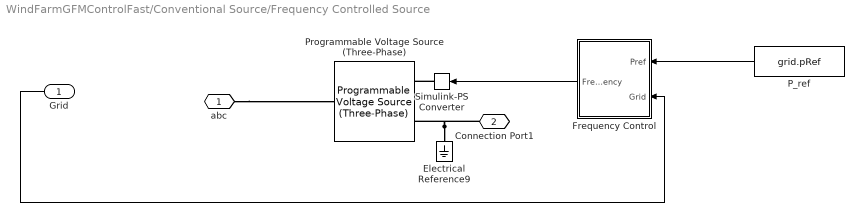
== system WindFarmGFMControlFast/Conventional Source/Frequency Controlled Source ==
  Grid : Inport
  Electrical Reference9 : fl_lib/Electrical/Electrical Elements/Electrical Reference
  Frequency Control : Subsystem
  P_ref : Constant  Value=grid.pRef
  Programmable Voltage Source (Three-Phase) : ee_lib/Sources/Programmable Voltage Source (Three-Phase)  magnitude_type=ee.enum.timechanging.constant  vline_rms=grid.voltage V  magn_ramp=1 V/s  magn_step=1 V  magn_modu_magn=1 V  magn_modu_freq=1 Hz  magn_t1=1 s  magn_t2=2 s  frequency_type=ee.enum.timechanging.external  freq=60 Hz  freq_ramp=1 Hz/s  freq_step=1 Hz  freq_modu_magn=1 Hz  freq_modu_freq=1 Hz  freq_t1=1 s  freq_t2=2 s  phase_type=ee.enum.timechanging.constant  shift=0 deg  phase_ramp=1 deg/s  phase_step=1 deg  phase_modu_magn=1 deg  phase_modu_freq=1 Hz  phase_t1=1 s  phase_t2=2 s  impedance_option=4  SShortCircuit=1e6 A*V  XR=15  R=grid.rs Ohm  L=grid.ls mH  G_parasitic=1e-6 1/Ohm  harmonic_option=0  harmonic_orders=[5, 7, 11, 13]  harmonic_ratios=[.1, .1, .1, .1]  harmonic_shifts=[0, 0, 0, 0] deg  harmonic_sequences=[1, 1, 1, 1]  harmonic_t1=-inf s  harmonic_t2=inf s  I_specify=off  I_priority=None  I=[0, 0, 0] A  I_nominal_specify=off  I_nominal_unit=A  I_nominal_value=1  V_specify=off  V_priority=None  V=[0, 0, 0] V  V_nominal_specify=off  V_nominal_unit=V  V_nominal_value=1
      settings: InternalSimscapePortConfiguration="{\"Bottom\":[],\"Left\":[{\"id\":\"ext_freq\",\"label\":\"F\",\"type\":\"input\"},{\"id\":\"n\",\"label\":\"n\",\"type\":\"foundation.electrical.electrical\"}],\"Right\":[{\"id\":\"N\",\"label\":\"~\",\"type\":\"foundation.electrical.three_phase\"}],\"Top\":[]}"
  Simulink-PS Converter : nesl_utility/Simulink-PS Converter  PhysicalDomain=network_engine_domain  SubClassName=ps_input  LeftPortType=input  RightPortType=output  PseudoPeriodic=off  Frequencies=[]  NoiseDistribution=none  NoiseParameters=[]  Unit=1  AffineConversion=off  FilteringAndDerivatives=provide  SimscapeFilterOrder=1  InputFilterTimeConstant=0.001  UdotUserProvided=0
  abc : PMIOPort  Side=Right
  Connection Port1 : PMIOPort  Port=2  Side=Left
  wires:
  Grid/1 -> Frequency Control/2(Grid)
  P_ref/1 -> Frequency Control/1(Pref)
  Frequency Control/1(Frequency) -> Simulink-PS Converter/1
  connections:
  Electrical Reference9/LConn1 -- Connection Port1/RConn1 -- Programmable Voltage Source (Three-Phase)/LConn2
  Simulink-PS Converter/RConn1 -- Programmable Voltage Source (Three-Phase)/LConn1
  abc/RConn1 -- Programmable Voltage Source (Three-Phase)/RConn1

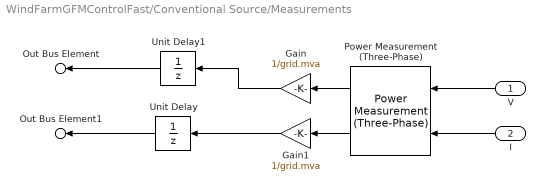
== system WindFarmGFMControlFast/Conventional Source/Measurements ==
  V : Inport
  I : Inport  Port=2
  Gain : Gain  Gain=1/grid.mva
  Gain1 : Gain  Gain=1/grid.mva
  Power Measurement (Three-Phase) : eePowerMeasurement/Power Measurement (Three-Phase)  LabelModeActiveChoice=Discrete  F=grid.frequency  K=[1]  Seq=Positive  Ts=Ts
  Unit Delay : UnitDelay  SampleTime=-1  HasFrameUpgradeWarning=on
  Unit Delay1 : UnitDelay  SampleTime=-1  HasFrameUpgradeWarning=on
  Out Bus Element : Outport  PortName=Grid  Element=Pe
  Out Bus Element1 : Outport  PortName=Grid  Element=Qe
  wires:
  Power Measurement (Three-Phase)/1 -> Gain/1
  I/1 -> Power Measurement (Three-Phase)/2
  Power Measurement (Three-Phase)/2 -> Gain1/1
  V/1 -> Power Measurement (Three-Phase)/1
  Gain/1 -> Unit Delay1/1
  Gain1/1 -> Unit Delay/1
  Unit Delay/1 -> Out Bus Element1/1
  Unit Delay1/1 -> Out Bus Element/1

== system WindFarmGFMControlFast/Fault1/CB1 ==
  Input : Inport
  Circuit Breaker Step off3 : ee_lib/Switches & Breakers/Circuit Breaker (Three-Phase)  R_closed=0.001 Ohm  G_open=1e-4 1/Ohm  threshold=0.5 V  breaker_behavior=ee.enum.switches.breakerBehavior.zeroCrossingDisable
      settings: InternalSimscapePortConfiguration="{\"Bottom\":[],\"Left\":[{\"id\":\"vT\",\"label\":\"vT\",\"type\":\"input\"},{\"id\":\"N1\",\"label\":\"~1\",\"type\":\"foundation.electrical.three_phase\"}],\"Right\":[{\"id\":\"N2\",\"label\":\"~2\",\"type\":\"foundation.electrical.three_phase\"}],\"Top\":[]}"
  Simulink-PS Converter3 : nesl_utility/Simulink-PS Converter  PhysicalDomain=network_engine_domain  SubClassName=ps_input  LeftPortType=input  RightPortType=output  PseudoPeriodic=off  Frequencies=[]  NoiseDistribution=none  NoiseParameters=[]  Unit=1  AffineConversion=off  FilteringAndDerivatives=zero  SimscapeFilterOrder=1  InputFilterTimeConstant=0.001  UdotUserProvided=1
  Conn2 : PMIOPort  Side=Left
  Conn1 : PMIOPort  Port=2  Side=Right
  wires:
  Input/1 -> Simulink-PS Converter3/1
  connections:
  Circuit Breaker Step off3/LConn2 -- Conn2/RConn1
  Circuit Breaker Step off3/LConn1 -- Simulink-PS Converter3/RConn1
  Circuit Breaker Step off3/RConn1 -- Conn1/RConn1

== system WindFarmGFMControlFast/Loads/CB1 ==
  Input : Inport
  Circuit Breaker Step off3 : ee_lib/Switches & Breakers/Circuit Breaker (Three-Phase)  R_closed=0.001 Ohm  G_open=1e-4 1/Ohm  threshold=0.5 V  breaker_behavior=ee.enum.switches.breakerBehavior.zeroCrossingDisable
      settings: InternalSimscapePortConfiguration="{\"Bottom\":[],\"Left\":[{\"id\":\"vT\",\"label\":\"vT\",\"type\":\"input\"},{\"id\":\"N1\",\"label\":\"~1\",\"type\":\"foundation.electrical.three_phase\"}],\"Right\":[{\"id\":\"N2\",\"label\":\"~2\",\"type\":\"foundation.electrical.three_phase\"}],\"Top\":[]}"
  Simulink-PS Converter3 : nesl_utility/Simulink-PS Converter  PhysicalDomain=network_engine_domain  SubClassName=ps_input  LeftPortType=input  RightPortType=output  PseudoPeriodic=off  Frequencies=[]  NoiseDistribution=none  NoiseParameters=[]  Unit=1  AffineConversion=off  FilteringAndDerivatives=zero  SimscapeFilterOrder=1  InputFilterTimeConstant=0.001  UdotUserProvided=1
  Conn2 : PMIOPort  Side=Left
  Conn1 : PMIOPort  Port=2  Side=Right
  wires:
  Input/1 -> Simulink-PS Converter3/1
  connections:
  Circuit Breaker Step off3/RConn1 -- Conn1/RConn1
  Circuit Breaker Step off3/LConn1 -- Simulink-PS Converter3/RConn1
  Circuit Breaker Step off3/LConn2 -- Conn2/RConn1

== system WindFarmGFMControlFast/PLL & Measurements/Measurement1 ==
  u : Inport
  Lead-Lag Filter1 : spsLeadLagFilterLib/Lead-Lag Filter  T1=0  T2=windController.tSensor  Vdc_Init=0  Ts=Ts
  Ig : Outport
  wires:
  Lead-Lag Filter1/1 -> Ig/1
  u/1 -> Lead-Lag Filter1/1

== system WindFarmGFMControlFast/PLL & Measurements/Measurement2 ==
  u : Inport
  Lead-Lag Filter1 : spsLeadLagFilterLib/Lead-Lag Filter  T1=0  T2=windController.tSensor  Vdc_Init=0  Ts=Ts
  Vg : Outport
  wires:
  Lead-Lag Filter1/1 -> Vg/1
  u/1 -> Lead-Lag Filter1/1

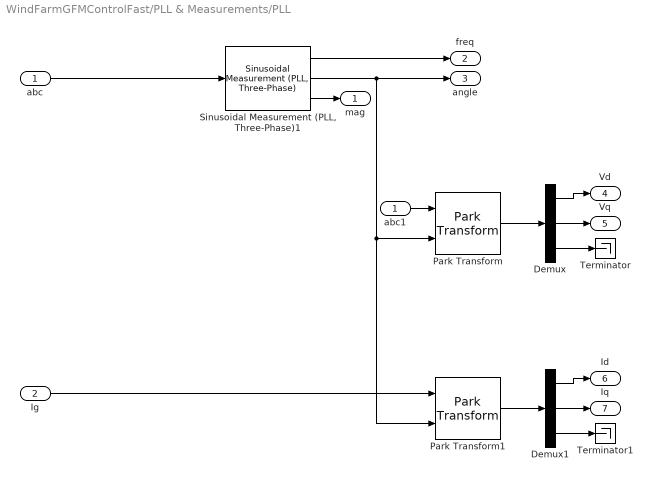
== system WindFarmGFMControlFast/PLL & Measurements/PLL ==
  abc : Inport
  Ig : Inport  Port=2
  Demux : Demux  Outputs=3
  Demux1 : Demux  Outputs=3
  Park Transform : eeTransforms/Park Transform  AxisAlignment=Q-axis  PowerInvariant=off
  Park Transform1 : eeTransforms/Park Transform  AxisAlignment=Q-axis  PowerInvariant=off
  "Sinusoidal Measurement (PLL, Three-Phase)1" : eeSinusoidalMeasurementV2/Sinusoidal Measurement (PLL, Three-Phase)  Kp_LF=pll.kp  Ki_LF=pll.ki  F0=grid.frequency  Theta0=0  Ts=Ts
      settings: LibrarySourceBlock=|
      | ee_sl_lib/Measurements/Sinusoidal Measurement
      | (PLL, Three-Phase)
  Terminator : Terminator
  Terminator1 : Terminator
  abc1 : InportShadow
  mag : Outport
  freq : Outport  Port=2
  angle : Outport  Port=3
  Vd : Outport  Port=4
  Vq : Outport  Port=5
  Id : Outport  Port=6
  Iq : Outport  Port=7
  wires:
  Demux/3 -> Terminator/1
  Park Transform/1 -> Demux/1
  Demux/1 -> Vd/1
  Demux/2 -> Vq/1
  "Sinusoidal Measurement (PLL, Three-Phase)1"/3 -> mag/1
  "Sinusoidal Measurement (PLL, Three-Phase)1"/2 -> angle/1, Park Transform/2, Park Transform1/2
  Ig/1 -> Park Transform1/1
  Demux1/2 -> Iq/1
  Park Transform1/1 -> Demux1/1
  Demux1/1 -> Id/1
  Demux1/3 -> Terminator1/1
  abc1/1 -> Park Transform/1
  abc/1 -> "Sinusoidal Measurement (PLL, Three-Phase)1"/1
  "Sinusoidal Measurement (PLL, Three-Phase)1"/1 -> freq/1

== system WindFarmGFMControlFast/Wind Farm/CB2 ==
  Input : Inport
  Circuit Breaker Step off3 : ee_lib/Switches & Breakers/Circuit Breaker (Three-Phase)  R_closed=0.001 Ohm  G_open=1e-4 1/Ohm  threshold=0.5 V  breaker_behavior=ee.enum.switches.breakerBehavior.zeroCrossingDisable
      settings: InternalSimscapePortConfiguration="{\"Bottom\":[],\"Left\":[{\"id\":\"vT\",\"label\":\"vT\",\"type\":\"input\"},{\"id\":\"N1\",\"label\":\"~1\",\"type\":\"foundation.electrical.three_phase\"}],\"Right\":[{\"id\":\"N2\",\"label\":\"~2\",\"type\":\"foundation.electrical.three_phase\"}],\"Top\":[]}"
  Simulink-PS Converter3 : nesl_utility/Simulink-PS Converter  PhysicalDomain=network_engine_domain  SubClassName=ps_input  LeftPortType=input  RightPortType=output  PseudoPeriodic=off  Frequencies=[]  NoiseDistribution=none  NoiseParameters=[]  Unit=1  AffineConversion=off  FilteringAndDerivatives=zero  SimscapeFilterOrder=1  InputFilterTimeConstant=0.001  UdotUserProvided=1
  Conn2 : PMIOPort  Side=Left
  Conn1 : PMIOPort  Port=2  Side=Right
  wires:
  Input/1 -> Simulink-PS Converter3/1
  connections:
  Circuit Breaker Step off3/RConn1 -- Conn1/RConn1
  Circuit Breaker Step off3/LConn1 -- Simulink-PS Converter3/RConn1
  Circuit Breaker Step off3/LConn2 -- Conn2/RConn1

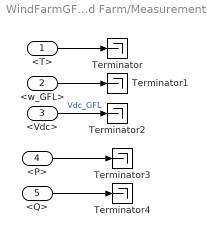
== system WindFarmGFMControlFast/Wind Farm/Measurements ==
  <T> : Inport
  <w_GFL> : Inport  Port=2
  <Vdc> : Inport  Port=3
  <P> : Inport  Port=4
  <Q> : Inport  Port=5
  Terminator{,1..4} (5 alike) : Terminator
  wires:
  <Vdc>/1 -> Terminator2/1  "Vdc_GFL"
  <Q>/1 -> Terminator4/1
  <w_GFL>/1 -> Terminator1/1
  <T>/1 -> Terminator/1
  <P>/1 -> Terminator3/1

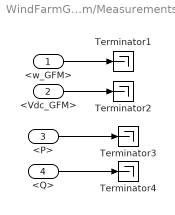
== system WindFarmGFMControlFast/Wind Farm/Measurements1 ==
  <w_GFM> : Inport
  <Vdc_GFM> : Inport  Port=2
  <P> : Inport  Port=3
  <Q> : Inport  Port=4
  Terminator{1..4} (4 alike) : Terminator
  wires:
  <P>/1 -> Terminator3/1
  <w_GFM>/1 -> Terminator1/1
  <Q>/1 -> Terminator4/1
  <Vdc_GFM>/1 -> Terminator2/1

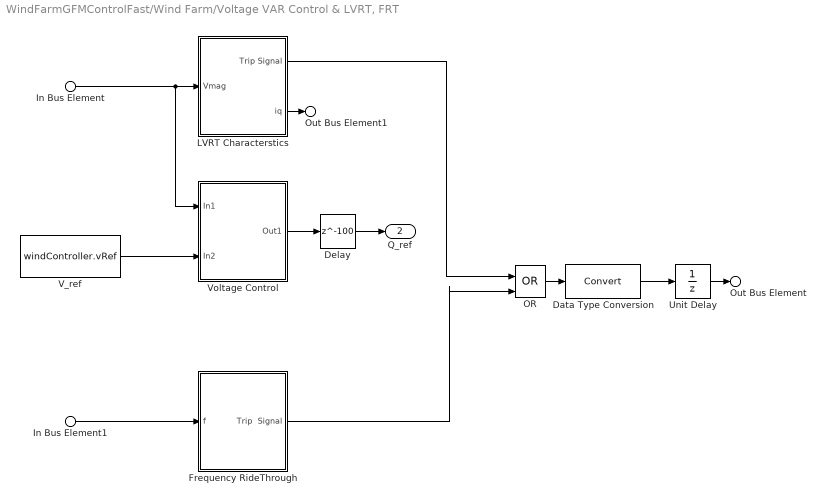
== system WindFarmGFMControlFast/Wind Farm/Voltage VAR Control & LVRT, FRT ==
  In Bus Element : Inport  PortName=Vbus  Element=Vmag
  In Bus Element1 : Inport  PortName=Vbus  Element=w
  Data Type Conversion : DataTypeConversion  RndMeth=Nearest  SaturateOnIntegerOverflow=off
  Delay : Delay  DelayLength=100
  Frequency RideThrough : Subsystem
  LVRT Characterstics : Subsystem
  OR : Logic  Operator=OR  IconShape=distinctive  AllPortsSameDT=off  OutDataTypeStr=boolean
  Unit Delay : UnitDelay  SampleTime=-1  HasFrameUpgradeWarning=on
  V_ref : Constant  Value=windController.vRef  SampleTime=Ts
  Voltage Control : Subsystem
  Out Bus Element : Outport  PortName=LVRT  Element=breaker
  Out Bus Element1 : Outport  PortName=LVRT  Element=iq
  Q_ref : Outport  Port=2
  wires:
  In Bus Element/1 -> LVRT Characterstics/1(Vmag), Voltage Control/1(In1)
  LVRT Characterstics/2(iq) -> Out Bus Element1/1
  V_ref/1 -> Voltage Control/2(In2)
  Voltage Control/1(Out1) -> Delay/1
  OR/1 -> Data Type Conversion/1
  LVRT Characterstics/1(Trip Signal) -> OR/1
  In Bus Element1/1 -> Frequency RideThrough/1(f)
  Data Type Conversion/1 -> Unit Delay/1
  Frequency RideThrough/1(Trip  Signal) -> OR/2
  Unit Delay/1 -> Out Bus Element/1
  Delay/1 -> Q_ref/1
